simulink model "robot2DOF_ContImpedancia_r2018b"  (R2018b)
settings: Solver=VariableStepAuto  StartTime=0.0  StopTime=10  MaxStep=0.01  MinStep=0.001  RelTol=1e-3
undefined symbols (not defined in the file or in its folder): coriolisAndCentripetal, dinamics, gravityCompensator, X, Y, Z
libraries: mblibv1 x19, sm_lib x11, nesl_utility x11
settings Model: Creator=raul  LastModifiedBy=raul
settings SimMechanicsCC: VisOnUpdateDiagram=on  VisDuringSimulation=on

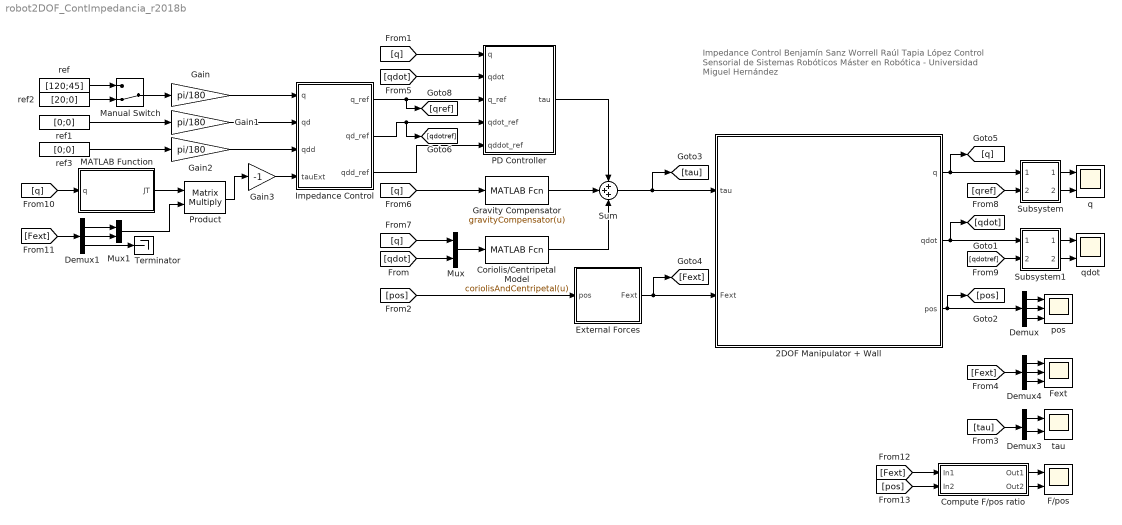
== system robot2DOF_ContImpedancia_r2018b ==
  note: Impedance Control
      | Benjamín Sanz Worrell
      | Raúl Tapia López
      |
      | Control Sensorial de Sistemas Robóticos
      | Máster en Robótica - Universidad Miguel Hernández
  2DOF Manipulator + Wall : Subsystem
      mask Display: image('manipulator_wall.png');
  Compute F/pos ratio : Subsystem
  "Coriolis/Centripetal Model " : MATLABFcn  MATLABFcn=coriolisAndCentripetal(u)
  Demux : Demux  Outputs=3
  Demux1 : Demux  Outputs=3
  Demux3 : Demux  Outputs=2
  Demux4 : Demux  Outputs=3
  External Forces : Subsystem
  F/pos : Scope  NumInputPorts=2
  Fext : Scope  NumInputPorts=3
  Gain : Gain  Gain=pi/180
  Gain1 : Gain  Gain=pi/180
  Gain2 : Gain  Gain=pi/180
  Gain3 : Gain  Gain=-1
  Gravity Compensator : MATLABFcn  MATLABFcn=gravityCompensator(u)
  Impedance Control : Subsystem
  MATLAB Function : MATLAB Function  TreatAsAtomicUnit=on
  Manual Switch : ManualSwitch  CurrentSetting=0
  Mux : Mux  Inputs=2
  Mux1 : Mux  Inputs=2
  PD Controller : Subsystem
  Product : Product  Multiplication=Matrix(*)  RndMeth=Zero
  Subsystem : Subsystem
  Subsystem1 : Subsystem
  Sum : Sum  Inputs=+++
  Terminator : Terminator
  pos : Scope  NumInputPorts=3
  q : Scope  NumInputPorts=2
  qdot : Scope  NumInputPorts=2
  ref : Constant  Value=[120;45]
  ref1 : Constant  Value=[0;0]
  ref2 : Constant  Value=[20;0]
  ref3 : Constant  Value=[0;0]
  tau : Scope  NumInputPorts=2
  wires:
  Demux/1 -> pos/1
  Demux/2 -> pos/2
  Demux/3 -> pos/3
  2DOF Manipulator + Wall/3(pos) -> Demux/1, [pos]
  2DOF Manipulator + Wall/1(q) -> [q], Subsystem/1(In1)
  Demux3/1 -> tau/1
  Demux3/2 -> tau/2
  Demux4/3 -> Fext/3
  Demux4/2 -> Fext/2
  Demux4/1 -> Fext/1
  Sum/1 -> [tau], 2DOF Manipulator + Wall/1(tau)
  Gravity Compensator/1 -> Sum/2
  [qdot] -> Mux/2
  Mux/1 -> "Coriolis/Centripetal Model "/1
  [q] -> PD Controller/1(q)
  "Coriolis/Centripetal Model "/1 -> Sum/3
  [tau] -> Demux3/1
  [Fext] -> Demux4/1
  [q] -> Gravity Compensator/1
  [qdot] -> PD Controller/2(qdot)
  PD Controller/1(tau) -> Sum/1
  [qref] -> Subsystem/2(In2)
  Subsystem/2(Out2) -> q/2
  Subsystem/1(Out1) -> q/1
  [qdotref] -> Subsystem1/2(In2)
  2DOF Manipulator + Wall/2(qdot) -> [qdot], Subsystem1/1(In1)
  Subsystem1/1(Out1) -> qdot/1
  Subsystem1/2(Out2) -> qdot/2
  Gain1/1 -> Impedance Control/2(qd)
  ref2/1 -> Manual Switch/2
  Gain/1 -> Impedance Control/1(q)
  ref/1 -> Manual Switch/1
  ref1/1 -> Gain1/1
  Manual Switch/1 -> Gain/1
  Impedance Control/1(q_ref) -> [qref], PD Controller/3(q_ref)
  Impedance Control/2(qd_ref) -> [qdotref], PD Controller/4(qdot_ref)
  Impedance Control/3(qdd_ref) -> PD Controller/5(qddot_ref)
  Gain2/1 -> Impedance Control/3(qdd)
  ref3/1 -> Gain2/1
  [q] -> MATLAB Function/1(q)
  MATLAB Function/1(JT) -> Product/1
  Gain3/1 -> Impedance Control/4(tauExt)
  [Fext] -> Demux1/1
  Demux1/2 -> Mux1/2
  Demux1/1 -> Mux1/1
  Mux1/1 -> Product/2
  Demux1/3 -> Terminator/1
  [pos] -> External Forces/1(pos)
  [q] -> Mux/1
  External Forces/1(Fext) -> [Fext], 2DOF Manipulator + Wall/2(Fext)
  Product/1 -> Gain3/1
  [Fext] -> Compute F/pos ratio/1(In1)
  [pos] -> Compute F/pos ratio/2(In2)
  Compute F/pos ratio/1(Out1) -> F/pos/1
  Compute F/pos ratio/2(Out2) -> F/pos/2

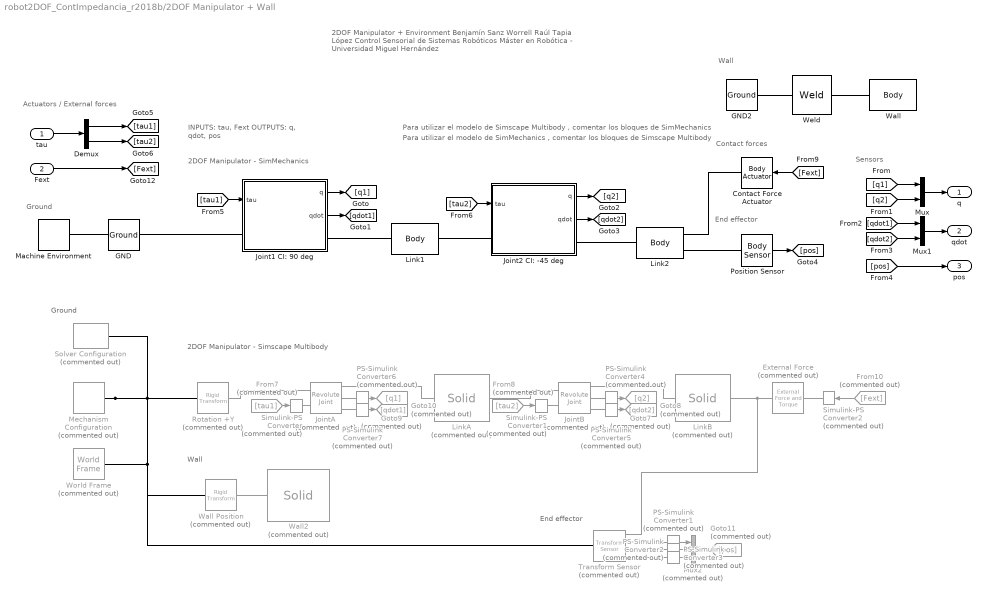
== system robot2DOF_ContImpedancia_r2018b/2DOF Manipulator + Wall ==
  note: Wall
  note: Wall
  note: Contact forces
  note: Para utilizar el modelo de Simscape Multibody , comentar los bloques de SimMechanics
  note: End effector
  note: INPUTS: tau, Fext
      | OUTPUTS: q, qdot, pos
  note: Actuators / External forces
  note: 2DOF Manipulator - SimMechanics
  note: Ground
  note: Sensors
  note: 2DOF Manipulator - Simscape Multibody
  note: End effector
  note: Ground
  note: Para utilizar el modelo de SimMechanics , comentar los bloques de Simscape Multibody
  note: 2DOF Manipulator + Environment
      | Benjamín Sanz Worrell
      | Raúl Tapia López
      |
      | Control Sensorial de Sistemas Robóticos
      | Máster en Robótica - Universidad Miguel Hernández
  tau : Inport
  Fext : Inport  Port=2
  Contact Force Actuator : mblibv1/Sensors &  Actuators/Body Actuator  UpdateFromCAD=off  PhysicalDomain=Mechanical  PortType=blob  ActuationStyle=Force  AngleUnits=deg  ArcVelocityUnits=deg/s  ArcAccelerationUnits=deg/s^2  CoordPositionUnits=m  VelocityUnits=m/s  AccelerationUnits=m/s^2  ForceUnits=N  TorqueUnits=N-m  ActiveIO=on  Width=3  DialogClass=MechanicalActuatorBlock  ReferenceFrame=Absolute (World)  Angle=off  CoordPosition=on  Force=on  Torque=off
      settings: SourceProductName=Simscape Multibody  SourceProductBaseCode=MS
  Demux : Demux  Outputs=2
  External Force : sm_lib/Forces and Torques/External Force and Torque  Commented=on  ForceResolutionFrame=AttachedFrame  EnableForceX=off  EnableForceY=off  EnableForceZ=off  EnableForce=on  TorqueResolutionFrame=AttachedFrame  EnableTorqueX=off  EnableTorqueY=off  EnableTorqueZ=off  EnableTorque=off
  From10 : From  Commented=on  GotoTag=Fext
  From7 : From  Commented=on  GotoTag=tau1
  From8 : From  Commented=on  GotoTag=tau2
  GND : mblibv1/Bodies/Ground  UpdateFromCAD=off  LeftPortType=env  RightPortType=workingframe  PhysicalDomain=Mechanical  DialogClass=GroundBlock  CoordPosition=[0 0 0]  CoordPositionUnits=m  StateVectorMgrId=18  MachineId=[9 0]  ShowEnvPort=on  ParameterChecksum=[2605844096, 4209328193, 971177056, 2557648036]  TopologyChecksum=[2062803494, 2049083245, 3945456521, 2961335378]
      settings: SourceProductName=Simscape  SourceProductBaseCode=SS
  GND2 : mblibv1/Bodies/Ground  UpdateFromCAD=off  LeftPortType=env  RightPortType=workingframe  PhysicalDomain=Mechanical  DialogClass=GroundBlock  CoordPosition=[0.3 0 0]  CoordPositionUnits=m  StateVectorMgrId=19  MachineId=[9 1]  ShowEnvPort=off  ParameterChecksum=[2106921359, 3945686204, 4148824445, 573166841]  TopologyChecksum=[551590820, 4054414437, 322053344, 2372914670]
      settings: SourceProductName=Simscape Multibody  SourceProductBaseCode=MS
  Goto10 : Goto  Commented=on  GotoTag=qdot1
  Goto11 : Goto  Commented=on  GotoTag=pos
  Goto7 : Goto  Commented=on  GotoTag=q2
  Goto8 : Goto  Commented=on  GotoTag=qdot2
  Goto9 : Goto  Commented=on  GotoTag=q1
  Joint1 CI: 90 deg : Subsystem
      mask Display: image('revolute.png');
  Joint2 CI: -45 deg : Subsystem
      mask Display: image('revolute.png');
  JointA : sm_lib/Joints/Revolute Joint  Commented=on  SenseConstraintForce=off  SenseConstraintForceX=off  SenseConstraintForceY=off  SenseConstraintForceZ=off  SenseConstraintTorque=off  SenseConstraintTorqueX=off  SenseConstraintTorqueY=off  SenseConstraintTorqueZ=off  SenseTotalForce=off  SenseTotalForceX=off  SenseTotalForceY=off  SenseTotalForceZ=off  SenseTotalTorque=off  SenseTotalTorqueX=off  SenseTotalTorqueY=off  SenseTotalTorqueZ=off  CompositeWrenchDir=FollowerOnBase  CompositeWrenchFrame=BaseFrame  EquilibriumPosition=0  EquilibriumPositionUnits=deg  SpringStiffness=0  SpringStiffnessUnits=N*m/deg  DampingCoefficient=0  DampingCoefficientUnits=N*m/(deg/s)  TorqueActuationMode=InputTorque  MotionActuationMode=ComputedMotion  SensePosition=on  SenseVelocity=on  SenseAcceleration=off  SenseTorqueForce=off  PositionTargetSpecify=on  PositionTargetPriority=High  PositionTargetValue=60  PositionTargetValueUnits=deg  VelocityTargetSpecify=off  VelocityTargetPriority=High  VelocityTargetValue=0  VelocityTargetValueUnits=deg/s
  JointB : sm_lib/Joints/Revolute Joint  Commented=on  SenseConstraintForce=off  SenseConstraintForceX=off  SenseConstraintForceY=off  SenseConstraintForceZ=off  SenseConstraintTorque=off  SenseConstraintTorqueX=off  SenseConstraintTorqueY=off  SenseConstraintTorqueZ=off  SenseTotalForce=off  SenseTotalForceX=off  SenseTotalForceY=off  SenseTotalForceZ=off  SenseTotalTorque=off  SenseTotalTorqueX=off  SenseTotalTorqueY=off  SenseTotalTorqueZ=off  CompositeWrenchDir=FollowerOnBase  CompositeWrenchFrame=BaseFrame  EquilibriumPosition=0  EquilibriumPositionUnits=deg  SpringStiffness=0  SpringStiffnessUnits=N*m/deg  DampingCoefficient=0  DampingCoefficientUnits=N*m/(deg/s)  TorqueActuationMode=InputTorque  MotionActuationMode=ComputedMotion  SensePosition=on  SenseVelocity=on  SenseAcceleration=off  SenseTorqueForce=off  PositionTargetSpecify=off  PositionTargetPriority=High  PositionTargetValue=60  PositionTargetValueUnits=deg  VelocityTargetSpecify=off  VelocityTargetPriority=High  VelocityTargetValue=0  VelocityTargetValueUnits=deg/s
  Link1 : mblibv1/Bodies/Body  LConnTagsString=CS1  RConnTagsString=CS2  UpdateFromCAD=off  DialogClass=MechanicalBodyBlock  Mass=10  MassUnits=kg  InertiaUnits=kg*m^2  Inertia=zeros(3,3)  Shape=Cylinder  ShapeDims=[1 1]  ShapeUnits=m  ShapeUse=false  Density=1  DensityUnits=kg/m^3  DensityUse=false  GraphicsMode=MACHINE_DEFAULT  BodyColorSelMode=MACHINE_DEFAULT  BodyColor=[1 0 0]  AttachedToCS=CG  CG=Left$CG$[0.2 0 0]$CS1$CS1$m$[0 0 0]$Euler X-Y-Z$deg$WORLD$false$none  WorkingFrames=Left$CS1$[0 0 0]$World$World$m$[0 0 0]$Euler X-Y-Z$deg$WORLD$true$none#Right$CS2$[0.2 0 0]$CS1$CS1$m$[0 0 0]$Euler X-Y-Z$deg$WORLD$true$none  CGPos=[0.2 0 0]  CGRot=[0 0 0]  CS0Pos=[]  CS0Rot=[]  CS1Pos=[0 0 0]  CS1Rot=[0 0 0]  CS2Pos=[0.2 0 0]  CS2Rot=[0 0 0]  CS3Pos=[]  CS3Rot=[]  CS4Pos=[]  CS4Rot=[]  CS5Pos=[]  CS5Rot=[]  CS6Pos=[]  CS6Rot=[]  CS7Pos=[]  CS7Rot=[]  CS8Pos=[]  CS8Rot=[]  CS9Pos=[]  CS9Rot=[]  CS10Pos=[]  CS10Rot=[]  CS11Pos=[]  CS11Rot=[]  CS12Pos=[]  CS12Rot=[]  CS13Pos=[]  CS13Rot=[]  CS14Pos=[]  CS14Rot=[]  CS15Pos=[]  CS15Rot=[]  CS16Pos=[]  CS16Rot=[]  CS17Pos=[]  CS17Rot=[]  CS18Pos=[]  CS18Rot=[]  CS19Pos=[]  CS19Rot=[]  CS20Pos=[]  CS20Rot=[]
      settings: SourceProductName=Simscape  SourceProductBaseCode=SS
  Link2 : mblibv1/Bodies/Body  LConnTagsString=CS1  RConnTagsString=CS3|CS2  UpdateFromCAD=off  DialogClass=MechanicalBodyBlock  Mass=10  MassUnits=kg  InertiaUnits=kg*m^2  Inertia=zeros(3,3)  Shape=Cylinder  ShapeDims=[1 1]  ShapeUnits=m  ShapeUse=false  Density=1  DensityUnits=kg/m^3  DensityUse=false  GraphicsMode=MACHINE_DEFAULT  BodyColorSelMode=MACHINE_DEFAULT  BodyColor=[1 0 0]  AttachedToCS=CG  CG=Left$CG$[0.2 0 0]$CS1$CS1$m$[0 0 0]$Euler X-Y-Z$deg$WORLD$false$none  WorkingFrames=Right$CS3$[0.2 0 0]$CS1$CS1$m$[0 0 0]$Euler X-Y-Z$deg$WORLD$true$none#Left$CS1$[0 0 0]$Adjoining$Adjoining$m$[0 0 0]$Euler X-Y-Z$deg$WORLD$true$none#Right$CS2$[0.2 0 0]$CS1$CS1$m$[0 0 0]$Euler X-Y-Z$deg$WORLD$true$none  CGPos=[0.2 0 0]  CGRot=[0 0 0]  CS0Pos=[]  CS0Rot=[]  CS1Pos=[0 0 0]  CS1Rot=[0 0 0]  CS2Pos=[0.2 0 0]  CS2Rot=[0 0 0]  CS3Pos=[0.2 0 0]  CS3Rot=[0 0 0]  CS4Pos=[]  CS4Rot=[]  CS5Pos=[]  CS5Rot=[]  CS6Pos=[]  CS6Rot=[]  CS7Pos=[]  CS7Rot=[]  CS8Pos=[]  CS8Rot=[]  CS9Pos=[]  CS9Rot=[]  CS10Pos=[]  CS10Rot=[]  CS11Pos=[]  CS11Rot=[]  CS12Pos=[]  CS12Rot=[]  CS13Pos=[]  CS13Rot=[]  CS14Pos=[]  CS14Rot=[]  CS15Pos=[]  CS15Rot=[]  CS16Pos=[]  CS16Rot=[]  CS17Pos=[]  CS17Rot=[]  CS18Pos=[]  CS18Rot=[]  CS19Pos=[]  CS19Rot=[]  CS20Pos=[]  CS20Rot=[]
      settings: SourceProductName=Simscape  SourceProductBaseCode=SS
  LinkA : sm_lib/Body Elements/Solid  Commented=on  InertiaType=PointMass  Mass=10  MassUnits=kg  CenterOfMass=[0 0 0]  CenterOfMassUnits=m  MomentsOfInertia=[1 1 1]  MomentsOfInertiaUnits=kg*m^2  ProductsOfInertia=[0 0 0]  ProductsOfInertiaUnits=kg*m^2  BasedOnType=Density  Density=1000  DensityUnits=kg/m^3  DoExposeReferenceFrame=off  SerializedFrames=<Frames><Frame><Id>Frame1</Id><Value><Name>F</Name><Origin><Source>GeometricFeature</Source><FeatureName>+y surface</FeatureName></Origin><PrimaryAxis><DefinedDirection>+Z</DefinedDirection><Source>ReferenceFrame</Source><SourceDirection>+Z</SourceDirection><FeatureName></FeatureName></PrimaryAxis><SecondaryAxis><DefinedDirection>+X</DefinedDirection><Source>ReferenceFrame</Source><SourceDirection>+X</SourceDirection><FeatureName></FeatureName></SecondaryAxis></Value></Frame><Frame><Id>Frame2</Id><Value><Name>B</Name><Origin><Source>GeometricFeature</Source><FeatureName>-y surface</FeatureName></Origin><PrimaryAxis><DefinedDirection>+Z</DefinedDirection><Source>ReferenceFrame</Source><SourceDirection>+Z</SourceDirection><FeatureName></FeatureName></PrimaryAxis><SecondaryAxis><DefinedDirection>+X</DefinedDirection><Source>ReferenceFrame</Source><SourceDirection>+X</SourceDirection><FeatureName></FeatureName></SecondaryAxis></Value></Frame></Frames>  GraphicType=FromGeometry  MarkerShape=Sphere  MarkerSize=10  GraphicVisPropType=SimpleVisualProperties  GraphicDiffuseColor=[0.5 0.5 0.5]  GraphicSpecularColor=[0.5 0.5 0.5 1.0]  GraphicAmbientColor=[0.15 0.15 0.15 1.0]  GraphicEmissiveColor=[0.0 0.0 0.0 1.0]  GraphicShininess=75  GraphicOpacity=1.0  GeometryShape=Brick  RectangleSize=[1 1]  RectangleSizeUnits=m  BrickDimensions=[0.01 0.2 0.01]  BrickDimensionUnits=m  CylinderRadius=1  CylinderRadiusUnits=m  CylinderLength=1  CylinderLengthUnits=m  SphereRadius=1  SphereRadiusUnits=m  EllipsoidRadii=[1 1 1]  EllipsoidRadiiUnits=m  ExtrusionCrossSection=[1 1; -1 1; -1 -1; 1 -1]  ExtrusionCrossSectionUnits=m  ExtrusionLength=1  ExtrusionLengthUnits=m  PolygonNumSides=3  PolygonOuterRadius=1  PolygonOuterRadiusUnits=m  ExtGeomFileType=STEP  ExtGeomFileUnits=m  RevolutionCrossSection=[1 1; 1 -1; 2 -1; 2 1]  RevolutionCrossSectionUnits=m  RevolutionExtent=Full  RevolutionAngle=180  RevolutionAngleUnits=deg
  LinkB : sm_lib/Body Elements/Solid  Commented=on  InertiaType=PointMass  Mass=10  MassUnits=kg  CenterOfMass=[0 0 0]  CenterOfMassUnits=m  MomentsOfInertia=[1 1 1]  MomentsOfInertiaUnits=kg*m^2  ProductsOfInertia=[0 0 0]  ProductsOfInertiaUnits=kg*m^2  BasedOnType=Density  Density=1000  DensityUnits=kg/m^3  DoExposeReferenceFrame=off  SerializedFrames=<Frames><Frame><Id>Frame1</Id><Value><Name>F</Name><Origin><Source>GeometricFeature</Source><FeatureName>+y surface</FeatureName></Origin><PrimaryAxis><DefinedDirection>+Z</DefinedDirection><Source>ReferenceFrame</Source><SourceDirection>+Z</SourceDirection><FeatureName></FeatureName></PrimaryAxis><SecondaryAxis><DefinedDirection>+X</DefinedDirection><Source>ReferenceFrame</Source><SourceDirection>+X</SourceDirection><FeatureName></FeatureName></SecondaryAxis></Value></Frame><Frame><Id>Frame2</Id><Value><Name>B</Name><Origin><Source>GeometricFeature</Source><FeatureName>-y surface</FeatureName></Origin><PrimaryAxis><DefinedDirection>+Z</DefinedDirection><Source>ReferenceFrame</Source><SourceDirection>+Z</SourceDirection><FeatureName></FeatureName></PrimaryAxis><SecondaryAxis><DefinedDirection>+X</DefinedDirection><Source>ReferenceFrame</Source><SourceDirection>+X</SourceDirection><FeatureName></FeatureName></SecondaryAxis></Value></Frame></Frames>  GraphicType=FromGeometry  MarkerShape=Sphere  MarkerSize=10  GraphicVisPropType=SimpleVisualProperties  GraphicDiffuseColor=[0.5 0.5 0.5]  GraphicSpecularColor=[0.5 0.5 0.5 1.0]  GraphicAmbientColor=[0.15 0.15 0.15 1.0]  GraphicEmissiveColor=[0.0 0.0 0.0 1.0]  GraphicShininess=75  GraphicOpacity=1.0  GeometryShape=Brick  RectangleSize=[1 1]  RectangleSizeUnits=m  BrickDimensions=[0.01 0.2 0.01]  BrickDimensionUnits=m  CylinderRadius=1  CylinderRadiusUnits=m  CylinderLength=1  CylinderLengthUnits=m  SphereRadius=1  SphereRadiusUnits=m  EllipsoidRadii=[1 1 1]  EllipsoidRadiiUnits=m  ExtrusionCrossSection=[1 1; -1 1; -1 -1; 1 -1]  ExtrusionCrossSectionUnits=m  ExtrusionLength=1  ExtrusionLengthUnits=m  PolygonNumSides=3  PolygonOuterRadius=1  PolygonOuterRadiusUnits=m  ExtGeomFileType=STEP  ExtGeomFileUnits=m  RevolutionCrossSection=[1 1; 1 -1; 2 -1; 2 1]  RevolutionCrossSectionUnits=m  RevolutionExtent=Full  RevolutionAngle=180  RevolutionAngleUnits=deg
  Machine Environment : mblibv1/Bodies/Machine Environment  PortType=env  PhysicalDomain=Mechanical  DialogTemplateClass=MECH.MachineEnvironment  SyncWhenCopied=off  Gravity=[0 -9.81 0]  GravityUnits=m/s^2  GravityAsSignal=off  Dimensionality=Auto-detect  AnalysisType=Forward dynamics  LinearAssemblyTolerance=1e-3  LinearAssemblyToleranceUnits=m  AngularAssemblyTolerance=1e-3  AngularAssemblyToleranceUnits=rad  ConstraintSolverType=Stabilizing  ConstraintRelTolerance=1e-4  ConstraintAbsTolerance=1e-4  UseRobustSingularityHandling=off  RedundancyAnalysisToleranceType=Automatically select tolerance  RedundancyAnalysisTolerance=1e-14  StatePerturbationType=Fixed  PerturbationSize=1e-5  VisualizeMachine=on  BodyVisualizationType=Use model default body geometries  BodyColorSelMode=Use model default  DefaultBodyColor=[1 0 0]
      settings: SourceProductName=Simscape  SourceProductBaseCode=SS
  Mechanism Configuration : sm_lib/Utilities/Mechanism Configuration  Commented=on  UniformGravity=Constant  GravityVector=[0 0 -9.80665]  GravityUnits=m/s^2  LinearizationDelta=0.001
  Mux : Mux  Inputs=2
  Mux1 : Mux  Inputs=2
  Mux2 : Mux  Commented=on  Inputs=3
  PS-Simulink Converter{1..7} (7 alike) : nesl_utility/PS-Simulink Converter  Commented=on  PhysicalDomain=network_engine_domain  SubClassName=ps_output  LeftPortType=input  RightPortType=output  PseudoPeriodic=off  Frequencies=[]  Unit=1  AffineConversion=off
  Position Sensor : mblibv1/Sensors &  Actuators/Body Sensor  UpdateFromCAD=off  PhysicalDomain=Mechanical  PortType=blob  Muxed=on  Pose=off  Angle=on  AngleUnits=deg  ArcVelocity=off  ArcVelocityUnits=deg/s  ArcAcceleration=off  ArcAccelerationUnits=deg/s^2  CoordPosition=on  CoordPositionUnits=m  Velocity=off  VelocityUnits=m/s  Acceleration=off  AccelerationUnits=m/s^2  Quaternion=on  QuaternionDT=off  QuaternionDDT=off  QuaternionUnits=off  OutputVector=[1]  ActiveIO=on  Width=3  DialogClass=MechanicalSensorBlock  ReferenceFrame=Absolute (World)
      settings: SourceProductName=Simscape  SourceProductBaseCode=SS
  "Rotation +Y " : sm_lib/Frames and Transforms/Rigid Transform  Commented=on  TranslationMethod=None  TranslationStandardOffset=0  TranslationLengthUnit=m  TranslationStandardAxis=+Z  TranslationCartesianOffset=[0 -1 0]  TranslationROffset=0  TranslationROffsetUnits=m  TranslationZOffset=0  TranslationZOffsetUnits=m  TranslationThetaOffset=0  TranslationThetaOffsetUnits=deg  RotationMethod=StandardAxis  RotationAngleUnits=deg  RotationStandardAxis=+Y  RotationAngle=90  RotationArbitraryAxis=[0 0 1]  FollAlignAxisA=+X  BaseAlignAxisA=+Y  FollAlignAxisB=+Y  BaseAlignAxisB=+Z  RotationSequenceAxes=FollowerAxes  RotationSequence=XYX  RotationSequenceAngles=[0 0 0]  RotationSequenceAnglesUnits=deg  RotationMatrix=[0 0 -1; 0 1 0; 1 0 0]
  Simulink-PS Converter : nesl_utility/Simulink-PS Converter  Commented=on  PhysicalDomain=network_engine_domain  SubClassName=ps_input  LeftPortType=input  RightPortType=output  PseudoPeriodic=off  Frequencies=[]  NoiseDistribution=none  NoiseParameters=[]  Unit=1  AffineConversion=off  FilteringAndDerivatives=provide  SimscapeFilterOrder=1  InputFilterTimeConstant=0.001  UdotUserProvided=0
  Simulink-PS Converter1 : nesl_utility/Simulink-PS Converter  Commented=on  PhysicalDomain=network_engine_domain  SubClassName=ps_input  LeftPortType=input  RightPortType=output  PseudoPeriodic=off  Frequencies=[]  NoiseDistribution=none  NoiseParameters=[]  Unit=1  AffineConversion=off  FilteringAndDerivatives=provide  SimscapeFilterOrder=1  InputFilterTimeConstant=0.001  UdotUserProvided=0
  Simulink-PS Converter2 : nesl_utility/Simulink-PS Converter  Commented=on  PhysicalDomain=network_engine_domain  SubClassName=ps_input  LeftPortType=input  RightPortType=output  PseudoPeriodic=off  Frequencies=[]  NoiseDistribution=none  NoiseParameters=[]  Unit=1  AffineConversion=off  FilteringAndDerivatives=provide  SimscapeFilterOrder=1  InputFilterTimeConstant=0.001  UdotUserProvided=0
  Solver Configuration : nesl_utility/Solver Configuration  Commented=on  PhysicalDomain=network_engine_domain  SubClassName=solver  LeftPortType=input  RightPortType=generic  Tones=[]  Harmonics=[]  SimulateNoise=off  Profile=off  UseLocalSampling=off  EnableSwitchedLinearOptims=on  FrequencyDomain=off  UseCCode=off  RelTol=0.001  AbsTol=1e-06  MinStep=1e-09  ToWorkspace=off  RevertToSquareIcSolve=off  NumHomotopyIterations=100  PhasorMode=off  PhasorModeNumHarmonics=1  DoDC=on  ResidualTolerance=1e-09  UseLocalSolver=off  LocalSolverChoice=NE_BACKWARD_EULER_ADVANCER  LocalSolverSampleTime=0.001  DoFixedCost=off  MaxNonlinIter=3  MaxModeIter=2  LinearAlgebra=auto  EquationFormulation=NE_TIME_EF  DelaysMemoryBudget=1024  AutomaticFiltering=on  FilteringTimeConstant=0.001  PartitionStorageMethod=AS_NEEDED  PartitionMemoryBudget=1024
  Transform Sensor : sm_lib/Frames and Transforms/Transform Sensor  Commented=on  MeasurementFrame=World  SenseAngle=off  SenseAxis=off  SenseAngle1=off  SenseAngle2=off  SenseAngle3=off  SenseQ=off  SenseR=off  SenseOmegaX=off  SenseOmegaY=off  SenseOmegaZ=off  SenseOmega1=off  SenseOmega2=off  SenseOmega3=off  SenseQDot=off  SenseRDot=off  SenseAlphaX=off  SenseAlphaY=off  SenseAlphaZ=off  SenseAlpha1=off  SenseAlpha2=off  SenseAlpha3=off  SenseQDDot=off  SenseRDDot=off  SenseX=on  SenseY=on  SenseZ=on  SenseRad=off  SenseAzim=off  SenseDist=off  SenseInc=off  SenseXDot=off  SenseYDot=off  SenseZDot=off  SenseRadDot=off  SenseAzimDot=off  SenseDistDot=off  SenseIncDot=off  SenseXDDot=off  SenseYDDot=off  SenseZDDot=off  SenseRadDDot=off  SenseAzimDDot=off  SenseDistDDot=off  SenseIncDDot=off
  Wall : mblibv1/Bodies/Body  LConnTagsString=CS1  RConnTagsString=CS2  UpdateFromCAD=off  DialogClass=MechanicalBodyBlock  Mass=1  MassUnits=kg  InertiaUnits=kg*m^2  Inertia=eye(3)  Shape=Cylinder  ShapeDims=[1 1]  ShapeUnits=m  ShapeUse=false  Density=1  DensityUnits=kg/m^3  DensityUse=false  GraphicsMode=MACHINE_DEFAULT  BodyColorSelMode=MACHINE_DEFAULT  BodyColor=[1 0 0]  AttachedToCS=CG  CG=Left$CG$[0 0.5 0]$CS1$CS1$m$[0 0 0]$Euler X-Y-Z$deg$WORLD$false$none  WorkingFrames=Left$CS1$[0 0 0]$Adjoining$Adjoining$m$[0 0 0]$Euler X-Y-Z$deg$WORLD$true$none#Right$CS2$[0 1 0]$CS1$CS1$m$[0 0 0]$Euler X-Y-Z$deg$WORLD$true$none  CGPos=[0 0.5 0]  CGRot=[0 0 0]  CS0Pos=[]  CS0Rot=[]  CS1Pos=[0 0 0]  CS1Rot=[0 0 0]  CS2Pos=[0 1 0]  CS2Rot=[0 0 0]  CS3Pos=[]  CS3Rot=[]  CS4Pos=[]  CS4Rot=[]  CS5Pos=[]  CS5Rot=[]  CS6Pos=[]  CS6Rot=[]  CS7Pos=[]  CS7Rot=[]  CS8Pos=[]  CS8Rot=[]  CS9Pos=[]  CS9Rot=[]  CS10Pos=[]  CS10Rot=[]  CS11Pos=[]  CS11Rot=[]  CS12Pos=[]  CS12Rot=[]  CS13Pos=[]  CS13Rot=[]  CS14Pos=[]  CS14Rot=[]  CS15Pos=[]  CS15Rot=[]  CS16Pos=[]  CS16Rot=[]  CS17Pos=[]  CS17Rot=[]  CS18Pos=[]  CS18Rot=[]  CS19Pos=[]  CS19Rot=[]  CS20Pos=[]  CS20Rot=[]
      settings: SourceProductName=Simscape Multibody  SourceProductBaseCode=MS
  Wall Position : sm_lib/Frames and Transforms/Rigid Transform  Commented=on  TranslationMethod=Cartesian  TranslationStandardOffset=0  TranslationLengthUnit=m  TranslationStandardAxis=+Z  TranslationCartesianOffset=[0 0.3 0]  TranslationROffset=0  TranslationROffsetUnits=m  TranslationZOffset=0  TranslationZOffsetUnits=m  TranslationThetaOffset=0  TranslationThetaOffsetUnits=deg  RotationMethod=None  RotationAngleUnits=deg  RotationStandardAxis=+Z  RotationAngle=0.0  RotationArbitraryAxis=[0 0 1]  FollAlignAxisA=+X  BaseAlignAxisA=+Y  FollAlignAxisB=+Y  BaseAlignAxisB=+Z  RotationSequenceAxes=FollowerAxes  RotationSequence=XYX  RotationSequenceAngles=[0 0 0]  RotationSequenceAnglesUnits=deg  RotationMatrix=[1 0 0; 0 1 0; 0 0 1]
  Wall2 : sm_lib/Body Elements/Solid  Commented=on  InertiaType=CalculateFromGeometry  Mass=1  MassUnits=kg  CenterOfMass=[0 0 0]  CenterOfMassUnits=m  MomentsOfInertia=[1 1 1]  MomentsOfInertiaUnits=kg*m^2  ProductsOfInertia=[0 0 0]  ProductsOfInertiaUnits=kg*m^2  BasedOnType=Density  Density=1000  DensityUnits=kg/m^3  DoExposeReferenceFrame=on  SerializedFrames=<Frames/>  GraphicType=FromGeometry  MarkerShape=Sphere  MarkerSize=10  GraphicVisPropType=SimpleVisualProperties  GraphicDiffuseColor=[1.0 0.4 0.4]  GraphicSpecularColor=[0.5 0.5 0.5 1.0]  GraphicAmbientColor=[0.15 0.15 0.15 1.0]  GraphicEmissiveColor=[0.0 0.0 0.0 1.0]  GraphicShininess=75  GraphicOpacity=1.0  GeometryShape=Brick  RectangleSize=[1 1]  RectangleSizeUnits=m  BrickDimensions=[1 0.01 1]  BrickDimensionUnits=m  CylinderRadius=1  CylinderRadiusUnits=m  CylinderLength=1  CylinderLengthUnits=m  SphereRadius=1  SphereRadiusUnits=m  EllipsoidRadii=[1 1 1]  EllipsoidRadiiUnits=m  ExtrusionCrossSection=[1 1; -1 1; -1 -1; 1 -1]  ExtrusionCrossSectionUnits=m  ExtrusionLength=1  ExtrusionLengthUnits=m  PolygonNumSides=3  PolygonOuterRadius=1  PolygonOuterRadiusUnits=m  ExtGeomFileType=STEP  ExtGeomFileUnits=m  RevolutionCrossSection=[1 1; 1 -1; 2 -1; 2 1]  RevolutionCrossSectionUnits=m  RevolutionExtent=Full  RevolutionAngle=180  RevolutionAngleUnits=deg
  Weld : mblibv1/Joints/Weld  LConnTagsString=__newl0  RConnTagsString=__newr0  UpdateFromCAD=off  NumSAPorts=0  CutJoint=off  MarkAsCut=off  Primitives=weld  PrimitiveProps=W$World$[0 1 0]$weld  DialogClass=JointBlock  WAxis=[0 1 0]
      settings: SourceProductName=Simscape Multibody  SourceProductBaseCode=MS
  World Frame : sm_lib/Frames and Transforms/World Frame  Commented=on
  q : Outport
  qdot : Outport  Port=2
  pos : Outport  Port=3
  wires:
  Joint2 CI: -45 deg/2(qdot) -> [qdot2]
  Position Sensor/1 -> [pos]
  Mux1/1 -> qdot/1
  Joint1 CI: 90 deg/2(qdot) -> [qdot1]
  [q2] -> Mux/2
  [pos] -> pos/1
  Joint2 CI: -45 deg/1(q) -> [q2]
  Joint1 CI: 90 deg/1(q) -> [q1]
  Mux/1 -> q/1
  [qdot1] -> Mux1/1
  [qdot2] -> Mux1/2
  [q1] -> Mux/1
  tau/1 -> Demux/1
  Demux/1 -> [tau1]
  Demux/2 -> [tau2]
  [tau1] -> Joint1 CI: 90 deg/1(tau)
  [tau2] -> Joint2 CI: -45 deg/1(tau)
  PS-Simulink Converter5/1 -> Goto8/1
  PS-Simulink Converter2/1 -> Mux2/2
  PS-Simulink Converter4/1 -> Goto7/1
  PS-Simulink Converter1/1 -> Mux2/1
  From7/1 -> Simulink-PS Converter/1
  From8/1 -> Simulink-PS Converter1/1
  PS-Simulink Converter7/1 -> Goto10/1
  PS-Simulink Converter6/1 -> Goto9/1
  PS-Simulink Converter3/1 -> Mux2/3
  Mux2/1 -> Goto11/1
  Fext/1 -> [Fext]
  [Fext] -> Contact Force Actuator/1
  From10/1 -> Simulink-PS Converter2/1
  connections:
  Machine Environment/RConn1 -- GND/LConn1
  Link1/LConn1 -- Joint1 CI: 90 deg/RConn1
  GND/RConn1 -- Joint1 CI: 90 deg/LConn1
  Link1/RConn1 -- Joint2 CI: -45 deg/LConn1
  Link2/LConn1 -- Joint2 CI: -45 deg/RConn1
  Mechanism Configuration/RConn1 -- "Rotation +Y "/LConn1 -- Solver Configuration/RConn1 -- Wall Position/LConn1 -- Transform Sensor/LConn1 -- World Frame/RConn1
  Simulink-PS Converter/RConn1 -- JointA/LConn2
  Transform Sensor/RConn2 -- PS-Simulink Converter1/LConn1
  LinkB/RConn1 -- JointB/RConn1
  LinkA/RConn1 -- JointA/RConn1
  JointB/LConn1 -- LinkA/LConn1
  Transform Sensor/RConn4 -- PS-Simulink Converter3/LConn1
  Transform Sensor/RConn1 -- External Force/RConn1 -- LinkB/LConn1
  "Rotation +Y "/RConn1 -- JointA/LConn1
  Transform Sensor/RConn3 -- PS-Simulink Converter2/LConn1
  PS-Simulink Converter5/LConn1 -- JointB/RConn3
  Simulink-PS Converter1/RConn1 -- JointB/LConn2
  PS-Simulink Converter4/LConn1 -- JointB/RConn2
  PS-Simulink Converter6/LConn1 -- JointA/RConn2
  PS-Simulink Converter7/LConn1 -- JointA/RConn3
  Position Sensor/LConn1 -- Link2/RConn2
  Contact Force Actuator/RConn1 -- Link2/RConn1
  Weld/LConn1 -- GND2/RConn1
  Weld/RConn1 -- Wall/LConn1
  Wall Position/RConn1 -- Wall2/RConn1
  Simulink-PS Converter2/RConn1 -- External Force/LConn1

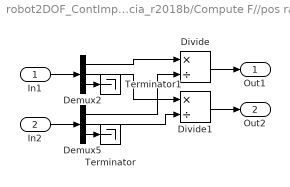
== system robot2DOF_ContImpedancia_r2018b/Compute F//pos ratio ==
  In1 : Inport
  In2 : Inport  Port=2
  Demux2 : Demux  Outputs=3
  Demux5 : Demux  Outputs=3
  Divide : Product  Inputs=*/
  Divide1 : Product  Inputs=*/
  Terminator : Terminator
  Terminator1 : Terminator
  Out1 : Outport
  Out2 : Outport  Port=2
  wires:
  In1/1 -> Demux2/1
  Demux5/1 -> Divide/2
  Demux5/2 -> Divide1/2
  Demux2/2 -> Divide1/1
  Divide1/1 -> Out2/1
  Demux2/1 -> Divide/1
  In2/1 -> Demux5/1
  Divide/1 -> Out1/1
  Demux5/3 -> Terminator/1
  Demux2/3 -> Terminator1/1

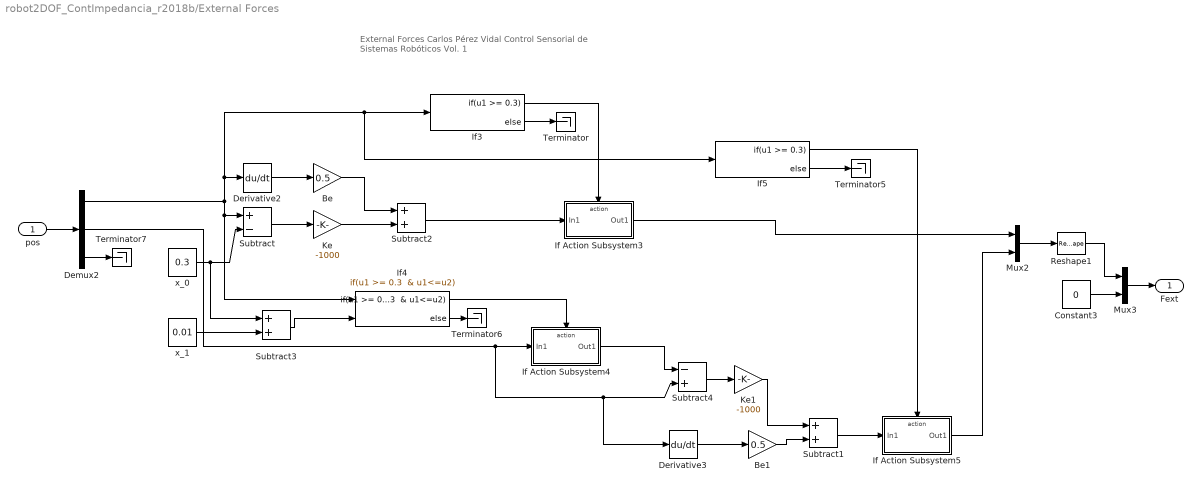
== system robot2DOF_ContImpedancia_r2018b/External Forces ==
  note: External Forces
      | Carlos Pérez Vidal
      | Control Sensorial de Sistemas Robóticos Vol. 1
  pos : Inport
  Be : Gain  Gain=0.5
  Be1 : Gain  Gain=0.5
  Constant3 : Constant  Value=0
  Demux2 : Demux  Outputs=3
  Derivative2 : Derivative
  Derivative3 : Derivative
  If Action Subsystem3 : Subsystem  TreatAsAtomicUnit=on
  If Action Subsystem4 : Subsystem  TreatAsAtomicUnit=on
  If Action Subsystem5 : Subsystem  TreatAsAtomicUnit=on
  If3 : If  IfExpression=u1 >= 0.3
  If4 : If  NumInputs=2  IfExpression="u1 >= 0.3  & u1<=u2"
  If5 : If  IfExpression=u1 >= 0.3
  Ke : Gain  Gain=-1000
  Ke1 : Gain  Gain=-1000
  Mux2 : Mux  Inputs=2
  Mux3 : Mux  Inputs=2
  Reshape1 : Reshape  OutputDimensionality=Column vector (2-D)
  Subtract : Sum  Inputs=+-
  Subtract1 : Sum
  Subtract2 : Sum
  Subtract3 : Sum
  Subtract4 : Sum  Inputs=-+
  Terminator{,5..7} (4 alike) : Terminator
  x_0 : Constant  Value=0.3
  x_1 : Constant  Value=0.01
  Fext : Outport
  wires:
  Subtract3/1 -> If4/2
  Be1/1 -> Subtract1/2
  If Action Subsystem4/1(Out1) -> Subtract4/1
  If5/2 -> Terminator5/1
  Mux2/1 -> Reshape1/1
  Reshape1/1 -> Mux3/1
  Subtract/1 -> Ke/1
  If4/2 -> Terminator6/1
  Ke/1 -> Subtract2/2
  Be/1 -> Subtract2/1
  x_0/1 -> Subtract/2, Subtract3/1
  Demux2/2 -> If Action Subsystem4/1(In1), Subtract4/2, Derivative3/1
  Derivative3/1 -> Be1/1
  Subtract2/1 -> If Action Subsystem3/1(In1)
  Demux2/3 -> Terminator7/1
  If3/1 -> If Action Subsystem3/Action
  If4/1 -> If Action Subsystem4/Action
  If5/1 -> If Action Subsystem5/Action
  Derivative2/1 -> Be/1
  Ke1/1 -> Subtract1/1
  If Action Subsystem3/1(Out1) -> Mux2/1
  x_1/1 -> Subtract3/2
  If Action Subsystem5/1(Out1) -> Mux2/2
  pos/1 -> Demux2/1
  If3/2 -> Terminator/1
  Demux2/1 -> Derivative2/1, If3/1, If5/1, Subtract/1, If4/1
  Subtract4/1 -> Ke1/1
  Subtract1/1 -> If Action Subsystem5/1(In1)
  Mux3/1 -> Fext/1
  Constant3/1 -> Mux3/2

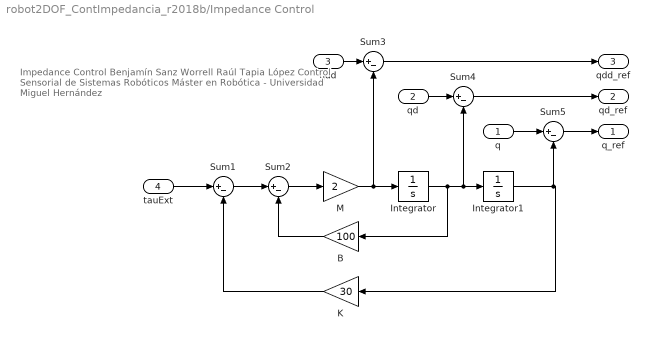
== system robot2DOF_ContImpedancia_r2018b/Impedance Control ==
  note: Impedance Control
      | Benjamín Sanz Worrell
      | Raúl Tapia López
      |
      | Control Sensorial de Sistemas Robóticos
      | Máster en Robótica - Universidad Miguel Hernández
  q : Inport
  qd : Inport  Port=2
  qdd : Inport  Port=3
  tauExt : Inport  Port=4
  B : Gain  Gain=100
  Integrator : Integrator
  Integrator1 : Integrator
  K : Gain  Gain=30
  M : Gain  Gain=2
  Sum{1..5} (5 alike) : Sum  Inputs=|+-
  q_ref : Outport
  qd_ref : Outport  Port=2
  qdd_ref : Outport  Port=3
  wires:
  q/1 -> Sum5/1
  Integrator1/1 -> K/1, Sum5/2
  Sum5/1 -> q_ref/1
  Integrator/1 -> Sum4/2, Integrator1/1, B/1
  M/1 -> Integrator/1, Sum3/2
  Sum2/1 -> M/1
  Sum1/1 -> Sum2/1
  B/1 -> Sum2/2
  K/1 -> Sum1/2
  tauExt/1 -> Sum1/1
  qd/1 -> Sum4/1
  Sum3/1 -> qdd_ref/1
  Sum4/1 -> qd_ref/1
  qdd/1 -> Sum3/1

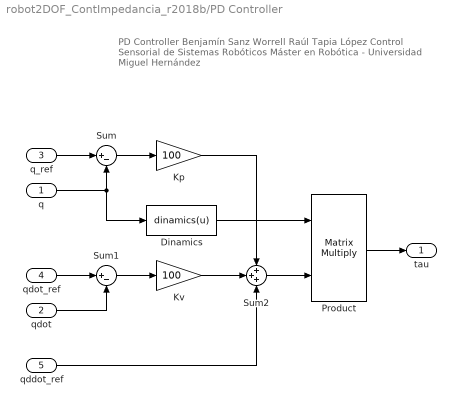
== system robot2DOF_ContImpedancia_r2018b/PD Controller ==
  note: PD Controller
      | Benjamín Sanz Worrell
      | Raúl Tapia López
      |
      | Control Sensorial de Sistemas Robóticos
      | Máster en Robótica - Universidad Miguel Hernández
  q : Inport
  qdot : Inport  Port=2
  q_ref : Inport  Port=3
  qdot_ref : Inport  Port=4
  qddot_ref : Inport  Port=5
  Dinamics : MATLABFcn  MATLABFcn=dinamics(u)  Output1D=off
  Kp : Gain  Gain=100
  Kv : Gain  Gain=100
  Product : Product  Multiplication=Matrix(*)  RndMeth=Zero
  Sum : Sum  Inputs=|+-
  Sum1 : Sum  Inputs=|+-
  Sum2 : Sum  Inputs=+++
  tau : Outport
  wires:
  Product/1 -> tau/1
  q_ref/1 -> Sum/1
  qdot_ref/1 -> Sum1/1
  Sum/1 -> Kp/1
  Sum1/1 -> Kv/1
  q/1 -> Dinamics/1, Sum/2
  Dinamics/1 -> Product/1
  Sum2/1 -> Product/2
  qdot/1 -> Sum1/2
  Kv/1 -> Sum2/2
  Kp/1 -> Sum2/1
  qddot_ref/1 -> Sum2/3

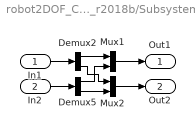
== system robot2DOF_ContImpedancia_r2018b/Subsystem ==
  In1 : Inport
  In2 : Inport  Port=2
  Demux2 : Demux  Outputs=2
  Demux5 : Demux  Outputs=2
  Mux1 : Mux  Inputs=2
  Mux2 : Mux  Inputs=2
  Out1 : Outport
  Out2 : Outport  Port=2
  wires:
  Demux2/1 -> Mux1/1
  In1/1 -> Demux2/1
  Mux1/1 -> Out1/1
  Demux5/1 -> Mux1/2
  Mux2/1 -> Out2/1
  In2/1 -> Demux5/1
  Demux2/2 -> Mux2/1
  Demux5/2 -> Mux2/2

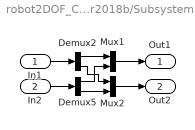
== system robot2DOF_ContImpedancia_r2018b/Subsystem1 ==
  In1 : Inport
  In2 : Inport  Port=2
  Demux2 : Demux  Outputs=2
  Demux5 : Demux  Outputs=2
  Mux1 : Mux  Inputs=2
  Mux2 : Mux  Inputs=2
  Out1 : Outport
  Out2 : Outport  Port=2
  wires:
  Demux2/1 -> Mux1/1
  In1/1 -> Demux2/1
  Mux1/1 -> Out1/1
  Demux5/1 -> Mux1/2
  Mux2/1 -> Out2/1
  In2/1 -> Demux5/1
  Demux2/2 -> Mux2/1
  Demux5/2 -> Mux2/2

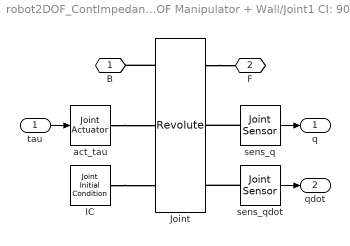
== system robot2DOF_ContImpedancia_r2018b/2DOF Manipulator + Wall/Joint1 CI: 90 deg ==
  tau : Inport
  IC : mblibv1/Sensors &  Actuators/Joint Initial Condition  UpdateFromCAD=off  LeftPortType=blob  RightPortType=blob  PhysicalDomain=mechanical  DialogClass=InitialConditionBlock  InitialConditions=P1$false$0$m$deg$0$m/s$deg/s#P2$false$0$m$deg$0$m/s$deg/s#P3$false$0$m$deg$0$m/s$deg/s#R1$true$90$m$deg$0$m/s$deg/s#R2$false$0$m$deg$0$m/s$deg/s#R3$false$0$m$deg$0$m/s$deg/s#S$false$0$m$deg$0$m/s$deg/s  P1PIC=0  P1VIC=0  P2PIC=0  P2VIC=0  P3PIC=0  P3VIC=0  R1PIC=90  R1VIC=0  R2PIC=0  R2VIC=0  R3PIC=0  R3VIC=0  SPIC=0  SVIC=0
      settings: SourceProductName=Simscape  SourceProductBaseCode=SS
  Joint : mblibv1/Joints/Revolute  LConnTagsString=__newl0|SA1|SA2  RConnTagsString=__newr0|SA1|SA2  UpdateFromCAD=off  NumSAPorts=4  CutJoint=off  MarkAsCut=off  Primitives=prismatic  PrimitiveProps=R1$World$[0 0 1]$revolute  DialogClass=JointBlock  R1Axis=[0 0 1]
      settings: SourceProductName=Simscape  SourceProductBaseCode=SS
  act_tau : mblibv1/Sensors &  Actuators/Joint Actuator  UpdateFromCAD=off  PhysicalDomain=Mechanical  PortType=blob  ActuationStyle=Force  AngleUnits=deg  ArcVelocityUnits=deg/s  ArcAccelerationUnits=deg/s^2  CoordPositionUnits=m  VelocityUnits=m/s  AccelerationUnits=m/s^2  ForceUnits=N  TorqueUnits=N*m  ActiveIO=on  Width=1  DialogClass=MechanicalActuatorBlock  Primitive=R1  ReferenceFrame=Absolute (World)
      settings: SourceProductName=Simscape  SourceProductBaseCode=SS
  sens_q : mblibv1/Sensors &  Actuators/Joint Sensor  UpdateFromCAD=off  PhysicalDomain=Mechanical  PortType=blob  Muxed=on  Pose=off  Angle=on  AngleUnits=rad  ArcVelocity=off  ArcVelocityUnits=deg/s  ArcAcceleration=off  ArcAccelerationUnits=deg/s^2  CoordPosition=on  CoordPositionUnits=m  Velocity=off  VelocityUnits=m/s  Acceleration=off  AccelerationUnits=m/s^2  Quaternion=on  QuaternionDT=off  QuaternionDDT=off  QuaternionUnits=off  OutputVector=[1]  ActiveIO=on  Width=1  DialogClass=MechanicalSensorBlock  Primitive=R1  Force=off  ForceUnits=N  Torque=off  TorqueUnits=N*m  ReferenceFrame=Absolute (World)  ReactionSensedSide=Base  ReactionReferenceFrame=Absolute (World)  ReactionForce=off  ReactionForceUnits=N  ReactionMoment=off  ReactionMomentUnits=N*m
      settings: SourceProductName=Simscape  SourceProductBaseCode=SS
  sens_qdot : mblibv1/Sensors &  Actuators/Joint Sensor  UpdateFromCAD=off  PhysicalDomain=Mechanical  PortType=blob  Muxed=on  Pose=off  Angle=off  AngleUnits=deg  ArcVelocity=on  ArcVelocityUnits=rad/s  ArcAcceleration=off  ArcAccelerationUnits=deg/s^2  CoordPosition=on  CoordPositionUnits=m  Velocity=off  VelocityUnits=m/s  Acceleration=off  AccelerationUnits=m/s^2  Quaternion=on  QuaternionDT=off  QuaternionDDT=off  QuaternionUnits=off  OutputVector=[1]  ActiveIO=on  Width=1  DialogClass=MechanicalSensorBlock  Primitive=R1  Force=off  ForceUnits=N  Torque=off  TorqueUnits=N*m  ReferenceFrame=Absolute (World)  ReactionSensedSide=Base  ReactionReferenceFrame=Absolute (World)  ReactionForce=off  ReactionForceUnits=N  ReactionMoment=off  ReactionMomentUnits=N*m
      settings: SourceProductName=Simscape  SourceProductBaseCode=SS
  B : PMIOPort  Side=Left
  F : PMIOPort  Port=2  Side=Right
  q : Outport
  qdot : Outport  Port=2
  wires:
  tau/1 -> act_tau/1
  sens_q/1 -> q/1
  sens_qdot/1 -> qdot/1
  connections:
  sens_qdot/LConn1 -- Joint/RConn3
  sens_q/LConn1 -- Joint/RConn2
  act_tau/RConn1 -- Joint/LConn2
  IC/RConn1 -- Joint/LConn3
  Joint/LConn1 -- B/RConn1
  Joint/RConn1 -- F/RConn1

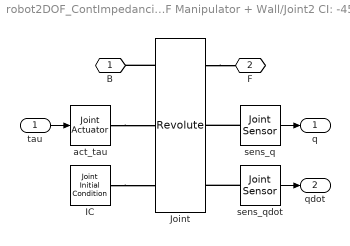
== system robot2DOF_ContImpedancia_r2018b/2DOF Manipulator + Wall/Joint2 CI: -45 deg ==
  tau : Inport
  IC : mblibv1/Sensors &  Actuators/Joint Initial Condition  UpdateFromCAD=off  LeftPortType=blob  RightPortType=blob  PhysicalDomain=mechanical  DialogClass=InitialConditionBlock  InitialConditions=P1$false$0$m$deg$0$m/s$deg/s#P2$false$0$m$deg$0$m/s$deg/s#P3$false$0$m$deg$0$m/s$deg/s#R1$true$-45$m$deg$0$m/s$deg/s#R2$false$0$m$deg$0$m/s$deg/s#R3$false$0$m$deg$0$m/s$deg/s#S$false$0$m$deg$0$m/s$deg/s  P1PIC=0  P1VIC=0  P2PIC=0  P2VIC=0  P3PIC=0  P3VIC=0  R1PIC=-45  R1VIC=0  R2PIC=0  R2VIC=0  R3PIC=0  R3VIC=0  SPIC=0  SVIC=0
      settings: SourceProductName=Simscape  SourceProductBaseCode=SS
  Joint : mblibv1/Joints/Revolute  LConnTagsString=__newl0|SA1|SA2  RConnTagsString=__newr0|SA1|SA2  UpdateFromCAD=off  NumSAPorts=4  CutJoint=off  MarkAsCut=off  Primitives=prismatic  PrimitiveProps=R1$World$[0 0 1]$revolute  DialogClass=JointBlock  R1Axis=[0 0 1]
      settings: SourceProductName=Simscape  SourceProductBaseCode=SS
  act_tau : mblibv1/Sensors &  Actuators/Joint Actuator  UpdateFromCAD=off  PhysicalDomain=Mechanical  PortType=blob  ActuationStyle=Force  AngleUnits=deg  ArcVelocityUnits=deg/s  ArcAccelerationUnits=deg/s^2  CoordPositionUnits=m  VelocityUnits=m/s  AccelerationUnits=m/s^2  ForceUnits=N  TorqueUnits=N-m  ActiveIO=on  Width=1  DialogClass=MechanicalActuatorBlock  Primitive=R1  ReferenceFrame=Absolute (World)
      settings: SourceProductName=Simscape  SourceProductBaseCode=SS
  sens_q : mblibv1/Sensors &  Actuators/Joint Sensor  UpdateFromCAD=off  PhysicalDomain=Mechanical  PortType=blob  Muxed=on  Pose=off  Angle=on  AngleUnits=rad  ArcVelocity=off  ArcVelocityUnits=deg/s  ArcAcceleration=off  ArcAccelerationUnits=deg/s^2  CoordPosition=on  CoordPositionUnits=m  Velocity=off  VelocityUnits=m/s  Acceleration=off  AccelerationUnits=m/s^2  Quaternion=on  QuaternionDT=off  QuaternionDDT=off  QuaternionUnits=off  OutputVector=[1]  ActiveIO=on  Width=1  DialogClass=MechanicalSensorBlock  Primitive=R1  Force=off  ForceUnits=N  Torque=off  TorqueUnits=N*m  ReferenceFrame=Absolute (World)  ReactionSensedSide=Base  ReactionReferenceFrame=Absolute (World)  ReactionForce=off  ReactionForceUnits=N  ReactionMoment=off  ReactionMomentUnits=N*m
      settings: SourceProductName=Simscape  SourceProductBaseCode=SS
  sens_qdot : mblibv1/Sensors &  Actuators/Joint Sensor  UpdateFromCAD=off  PhysicalDomain=Mechanical  PortType=blob  Muxed=on  Pose=off  Angle=off  AngleUnits=deg  ArcVelocity=on  ArcVelocityUnits=rad/s  ArcAcceleration=off  ArcAccelerationUnits=deg/s^2  CoordPosition=on  CoordPositionUnits=m  Velocity=off  VelocityUnits=m/s  Acceleration=off  AccelerationUnits=m/s^2  Quaternion=on  QuaternionDT=off  QuaternionDDT=off  QuaternionUnits=off  OutputVector=[1]  ActiveIO=on  Width=1  DialogClass=MechanicalSensorBlock  Primitive=R1  Force=off  ForceUnits=N  Torque=off  TorqueUnits=N*m  ReferenceFrame=Absolute (World)  ReactionSensedSide=Base  ReactionReferenceFrame=Absolute (World)  ReactionForce=off  ReactionForceUnits=N  ReactionMoment=off  ReactionMomentUnits=N*m
      settings: SourceProductName=Simscape  SourceProductBaseCode=SS
  B : PMIOPort  Side=Left
  F : PMIOPort  Port=2  Side=Right
  q : Outport
  qdot : Outport  Port=2
  wires:
  tau/1 -> act_tau/1
  sens_q/1 -> q/1
  sens_qdot/1 -> qdot/1
  connections:
  sens_qdot/LConn1 -- Joint/RConn3
  sens_q/LConn1 -- Joint/RConn2
  act_tau/RConn1 -- Joint/LConn2
  IC/RConn1 -- Joint/LConn3
  Joint/LConn1 -- B/RConn1
  Joint/RConn1 -- F/RConn1

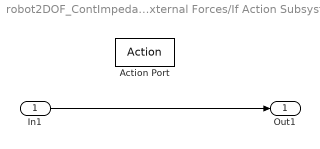
== system robot2DOF_ContImpedancia_r2018b/External Forces/If Action Subsystem3 ==
  In1 : Inport
  Action Port : ActionPort  ActionType=then
  Out1 : Outport
  wires:
  In1/1 -> Out1/1

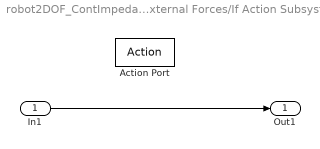
== system robot2DOF_ContImpedancia_r2018b/External Forces/If Action Subsystem4 ==
  In1 : Inport
  Action Port : ActionPort  ActionType=then
  Out1 : Outport
  wires:
  In1/1 -> Out1/1

== system robot2DOF_ContImpedancia_r2018b/External Forces/If Action Subsystem5 ==
  In1 : Inport
  Action Port : ActionPort  ActionType=then
  Out1 : Outport
  wires:
  In1/1 -> Out1/1

== matlab function robot2DOF_ContImpedancia_r2018b/MATLAB Function ==
  data: q input; JT output
% jacobianT.m
% Control Sensorial de Sistemas Robóticos
% Máster en Robótica - Universidad Miguel Hernández

function JT = jacobianT(q)

%%% Manipulator parameters
L1 = 0.2;
L2 = 0.2;

%%% Compute JT
J11 = -L2*sin(q(1)+q(2))-L1*sin(q(1));
J12 = -L2*sin(q(1)+q(2));
J21 = L2*cos(q(1)+q(2))+L1*cos(q(1));
J22 = L2*cos(q(1)+q(2));

JT = [J11 J12; J21 J22]';

end
